simulink model "MPCfastmpc"  (R2023a)
settings: Solver=ode4  StartTime=0.0  StopTime=tsim  FixedStep=baseRate  RelTol=1e-6  AbsTol=1e-6
values from neighbouring files (symbols this model uses):
  Ad = -C(7:12,4:9)    [theFastMPCSolver3.m]
  ALGORITHM = 7    [Run_Initializer.m]
  con0 = [n*N, 2*N, N, N, N]    [Run_Initializer.m]
  Gamma1_el = 0.12    [Run_Initializer.m]
  Gamma1_sh = 0.005    [Run_Initializer.m]
  Gamma1_wr = 0.025    [Run_Initializer.m]
  Gamma2_el = 5    [Run_Initializer.m]
  Gamma2_sh = 5    [Run_Initializer.m]
  Gamma2_wr = 5    [Run_Initializer.m]
  Gamma3_el = 10    [Run_Initializer.m]
  Gamma3_sh = 40    [Run_Initializer.m]
  Gamma3_wr = 40    [Run_Initializer.m]
  Gamma4_el = 0.039    [Run_Initializer.m]
  Gamma4_sh = 0.015    [Run_Initializer.m]
  Gamma4_wr = 0.029    [Run_Initializer.m]
  Gamma5_el = 800    [Run_Initializer.m]
  Gamma5_sh = 800    [Run_Initializer.m]
  Gamma5_wr = 800    [Run_Initializer.m]
  Gamma6_el = 0.000001    (= 1e-06)    [Run_Initializer.m]
  Gamma6_sh = 0.005    [Run_Initializer.m]
  Gamma6_wr = 0.02    [Run_Initializer.m]
  init_states_BLACK = [ct;thetat0].'    [Run_Initializer.m]
  init_states_BLUE = [pobj1;0].'    [Run_Initializer.m]
  init_states_RED = xi(1:3).'    [Run_Initializer.m]
  Kd_elarm = 0.8    [Run_Initializer.m]
  Kd_sharm = 1.0    (= 1)    [Run_Initializer.m]
  Kd_wrarm = 0.6    [Run_Initializer.m]
  Kp_elarm = 1.2    [Run_Initializer.m]
  Kp_sharm = 1.5    [Run_Initializer.m]
  Kp_wrarm = 2    [Run_Initializer.m]
  maxiterations = 10    [Run_Initializer.m]
  N = 15    [Run_Initializer.m]    (also in theFastMPCSolver3.m = length(z)/9)
  n = size(b,1)    [theFastMPCSolver3.m]
  Phi = 2*H + kappa*P.'*d2*P    [theFastMPCSolver3.m]
  Td = 2    [Run_Initializer.m]
  thetat_dot = 2.5 * d2r    (= 0.0436332312999)    [Run_Initializer.m]
  tol = 0.00015    [Run_Initializer.m]
  Tz_lim_elarm = .1    (= 0.1)    [Run_Initializer.m]
  Tz_lim_sharm = .1    (= 0.1)    [Run_Initializer.m]
  Tz_lim_wrarm = .1    (= 0.1)    [Run_Initializer.m]
  vobj1 = [0.00;0.00]    [Run_Initializer.m]
  vtar = [-0.005;0.005]    [Run_Initializer.m]
undefined symbols (not defined in the file or in its folder): a1, a2, a3, b0, b1, b2, b3, baseRate, cdockdeltax, cdockoa, Cmat, DiscIntNeverNeededParam, drop_states_ARM, drop_states_BLACK, drop_states_BLUE, drop_states_RED, ecoa, F_Black_X_nominal, F_Black_Y_nominal, F_Blue_X_nominal, F_Blue_Y_nominal, F_red_X_nominal, F_red_Y_nominal, F_thrusters_BLACK, F_thrusters_BLUE, F_thrusters_RED, Fmat, gamma, H, IBLACK, IBLUE, IDIST, IEE, IPROX, IRED, Kd_tb, Kd_tblue, Kd_tr, Kd_xb, Kd_xblue, Kd_xr, Kd_yb, Kd_yblue, Kd_yr, KOZ_actual, Kp_tb, Kp_tblue, Kp_tr, Kp_xb, Kp_xblue, Kp_xr, Kp_yb, Kp_yblue, Kp_yr, mBLACK, mBLUE, mDIST, mEE, mPROX, mRED ... (+29)
libraries: nvidiaSharedBlocks x8, simulink x8, dspsigops x6, dspstat3 x5, MainLibrary x4
(part 6 of 10)

== system MPCfastmpc/Phase #3: Experiment/Change BLUE Behavior/Sub-Phase #1/Custom Discrete PD (Attitude) ==
  ez : Inport
  Sum3 : Sum
  kd_tb : Gain  Gain=Kd_tblue
  kp_tb : Gain  Gain=Kp_tblue
  "x_dot -> x1" : Subsystem
  Tz : Outport  VectorParamsAs1DForOutWhenUnconnected=off
  wires:
  kd_tb/1 -> Sum3/1
  Sum3/1 -> Tz/1
  kp_tb/1 -> Sum3/2
  "x_dot -> x1"/1(dy(t)/dt) -> kd_tb/1
  ez/1 -> "x_dot -> x1"/1(y(t)), kp_tb/1

== system MPCfastmpc/Phase #3: Experiment/Change BLUE Behavior/Sub-Phase #1/Custom Discrete PD (X-Position) ==
  ex : Inport
  Sum3 : Sum
  kd_xb : Gain  Gain=Kd_xblue
  kp_xb : Gain  Gain=Kp_xblue
  "x_dot -> x1" : Subsystem
  Fx : Outport  VectorParamsAs1DForOutWhenUnconnected=off
  wires:
  kd_xb/1 -> Sum3/1
  ex/1 -> "x_dot -> x1"/1(y(t)), kp_xb/1
  kp_xb/1 -> Sum3/2
  "x_dot -> x1"/1(dy(t)/dt) -> kd_xb/1
  Sum3/1 -> Fx/1

== system MPCfastmpc/Phase #3: Experiment/Change BLUE Behavior/Sub-Phase #1/Custom Discrete PD (Y-Position) ==
  ey : Inport
  Sum3 : Sum
  kd_yb : Gain  Gain=Kd_yblue
  kp_yb : Gain  Gain=Kp_yblue
  "x_dot -> x1" : Subsystem
  Fy : Outport  VectorParamsAs1DForOutWhenUnconnected=off
  wires:
  kd_yb/1 -> Sum3/1
  Sum3/1 -> Fy/1
  kp_yb/1 -> Sum3/2
  "x_dot -> x1"/1(dy(t)/dt) -> kd_yb/1
  ey/1 -> "x_dot -> x1"/1(y(t)), kp_yb/1

== system MPCfastmpc/Phase #3: Experiment/Change BLUE Behavior/Sub-Phase #1/Hough Control ==
  Ref : Inport
  Act : Inport  Port=2
  MATLAB Function2 : MATLAB Function  TreatAsAtomicUnit=on
  MATLAB Function3 : MATLAB Function  TreatAsAtomicUnit=on
  MATLAB Function4 : MATLAB Function  TreatAsAtomicUnit=on
  Subtract2 : Sum  Inputs=+-
  Err : Outport  VectorParamsAs1DForOutWhenUnconnected=off
  wires:
  MATLAB Function4/1(e_out) -> Err/1
  MATLAB Function2/1(Oy) -> MATLAB Function4/1(Oy)
  Subtract2/1 -> MATLAB Function4/2(e_in)
  MATLAB Function2/2(Ox) -> Subtract2/1
  Act/1 -> MATLAB Function3/1(z)
  Ref/1 -> MATLAB Function2/1(z)
  MATLAB Function3/1(Ox) -> Subtract2/2

== system MPCfastmpc/Phase #3: Experiment/Change BLUE Behavior/Sub-Phase #2 /Custom Discrete PD (Attitude) ==
  ez : Inport
  Sum3 : Sum
  kd_tb : Gain  Gain=Kd_tblue
  kp_tb : Gain  Gain=Kp_tblue
  "x_dot -> x1" : Subsystem
  Tz : Outport  VectorParamsAs1DForOutWhenUnconnected=off
  wires:
  kd_tb/1 -> Sum3/1
  Sum3/1 -> Tz/1
  kp_tb/1 -> Sum3/2
  "x_dot -> x1"/1(dy(t)/dt) -> kd_tb/1
  ez/1 -> "x_dot -> x1"/1(y(t)), kp_tb/1

== system MPCfastmpc/Phase #3: Experiment/Change BLUE Behavior/Sub-Phase #2 /Custom Discrete PD (X-Position) ==
  ex : Inport
  Sum3 : Sum
  kd_xb : Gain  Gain=Kd_xblue
  kp_xb : Gain  Gain=Kp_xblue
  "x_dot -> x1" : Subsystem
  Fx : Outport  VectorParamsAs1DForOutWhenUnconnected=off
  wires:
  kd_xb/1 -> Sum3/1
  ex/1 -> "x_dot -> x1"/1(y(t)), kp_xb/1
  kp_xb/1 -> Sum3/2
  "x_dot -> x1"/1(dy(t)/dt) -> kd_xb/1
  Sum3/1 -> Fx/1

== system MPCfastmpc/Phase #3: Experiment/Change BLUE Behavior/Sub-Phase #2 /Custom Discrete PD (Y-Position) ==
  ey : Inport
  Sum3 : Sum
  kd_yb : Gain  Gain=Kd_yblue
  kp_yb : Gain  Gain=Kp_yblue
  "x_dot -> x1" : Subsystem
  Fy : Outport  VectorParamsAs1DForOutWhenUnconnected=off
  wires:
  kd_yb/1 -> Sum3/1
  Sum3/1 -> Fy/1
  kp_yb/1 -> Sum3/2
  "x_dot -> x1"/1(dy(t)/dt) -> kd_yb/1
  ey/1 -> "x_dot -> x1"/1(y(t)), kp_yb/1

== system MPCfastmpc/Phase #3: Experiment/Change BLUE Behavior/Sub-Phase #2 /Hough Control ==
  Ref : Inport
  Act : Inport  Port=2
  MATLAB Function2 : MATLAB Function  TreatAsAtomicUnit=on
  MATLAB Function3 : MATLAB Function  TreatAsAtomicUnit=on
  MATLAB Function4 : MATLAB Function  TreatAsAtomicUnit=on
  Subtract2 : Sum  Inputs=+-
  Err : Outport  VectorParamsAs1DForOutWhenUnconnected=off
  wires:
  MATLAB Function4/1(e_out) -> Err/1
  MATLAB Function2/1(Oy) -> MATLAB Function4/1(Oy)
  Subtract2/1 -> MATLAB Function4/2(e_in)
  MATLAB Function2/2(Ox) -> Subtract2/1
  Act/1 -> MATLAB Function3/1(z)
  Ref/1 -> MATLAB Function2/1(z)
  MATLAB Function3/1(Ox) -> Subtract2/2

== system MPCfastmpc/Phase #3: Experiment/Change BLUE Behavior/Sub-Phase #3 /Custom Discrete PD (Attitude) ==
  ez : Inport
  Sum3 : Sum
  kd_tb : Gain  Gain=Kd_tblue
  kp_tb : Gain  Gain=Kp_tblue
  "x_dot -> x1" : Subsystem
  Tz : Outport  VectorParamsAs1DForOutWhenUnconnected=off
  wires:
  kd_tb/1 -> Sum3/1
  Sum3/1 -> Tz/1
  kp_tb/1 -> Sum3/2
  "x_dot -> x1"/1(dy(t)/dt) -> kd_tb/1
  ez/1 -> "x_dot -> x1"/1(y(t)), kp_tb/1

== system MPCfastmpc/Phase #3: Experiment/Change BLUE Behavior/Sub-Phase #3 /Custom Discrete PD (X-Position) ==
  ex : Inport
  Sum3 : Sum
  kd_xb : Gain  Gain=Kd_xblue
  kp_xb : Gain  Gain=Kp_xblue
  "x_dot -> x1" : Subsystem
  Fx : Outport  VectorParamsAs1DForOutWhenUnconnected=off
  wires:
  kd_xb/1 -> Sum3/1
  ex/1 -> "x_dot -> x1"/1(y(t)), kp_xb/1
  kp_xb/1 -> Sum3/2
  "x_dot -> x1"/1(dy(t)/dt) -> kd_xb/1
  Sum3/1 -> Fx/1

== system MPCfastmpc/Phase #3: Experiment/Change BLUE Behavior/Sub-Phase #3 /Custom Discrete PD (Y-Position) ==
  ey : Inport
  Sum3 : Sum
  kd_yb : Gain  Gain=Kd_yblue
  kp_yb : Gain  Gain=Kp_yblue
  "x_dot -> x1" : Subsystem
  Fy : Outport  VectorParamsAs1DForOutWhenUnconnected=off
  wires:
  kd_yb/1 -> Sum3/1
  Sum3/1 -> Fy/1
  kp_yb/1 -> Sum3/2
  "x_dot -> x1"/1(dy(t)/dt) -> kd_yb/1
  ey/1 -> "x_dot -> x1"/1(y(t)), kp_yb/1

== system MPCfastmpc/Phase #3: Experiment/Change BLUE Behavior/Sub-Phase #3 /Hough Control ==
  Ref : Inport
  Act : Inport  Port=2
  MATLAB Function2 : MATLAB Function  TreatAsAtomicUnit=on
  MATLAB Function3 : MATLAB Function  TreatAsAtomicUnit=on
  MATLAB Function4 : MATLAB Function  TreatAsAtomicUnit=on
  Subtract2 : Sum  Inputs=+-
  Err : Outport  VectorParamsAs1DForOutWhenUnconnected=off
  wires:
  MATLAB Function4/1(e_out) -> Err/1
  MATLAB Function2/1(Oy) -> MATLAB Function4/1(Oy)
  Subtract2/1 -> MATLAB Function4/2(e_in)
  MATLAB Function2/2(Ox) -> Subtract2/1
  Act/1 -> MATLAB Function3/1(z)
  Ref/1 -> MATLAB Function2/1(z)
  MATLAB Function3/1(Ox) -> Subtract2/2

== system MPCfastmpc/Phase #3: Experiment/Change BLUE Behavior/Sub-Phase #3 /Subsystem ==
  Add : Sum
  Add1 : Sum  Inputs=+-
  Constant : Constant  Value=vobj1
  Constant1 : Constant  Value=init_states_BLUE(1)
  Constant2 : Constant  Value=Phase3_SubPhase2_End
  Data Store Read : DataStoreRead  DataStoreName=Univ_Time  IndexOptions=Index vector (dialog)  Indices=1  OutputSizes=1
  Demux : Demux  Outputs=2
  Product : Product
  Terminator : Terminator
  Out1 : Outport
  wires:
  Add/1 -> Out1/1
  Demux/2 -> Terminator/1
  Constant/1 -> Demux/1
  Constant1/1 -> Add/1
  Product/1 -> Add/2
  Demux/1 -> Product/1
  Constant2/1 -> Add1/2
  Data Store Read/1 -> Add1/1
  Add1/1 -> Product/2

== system MPCfastmpc/Phase #3: Experiment/Change BLUE Behavior/Sub-Phase #3 /Subsystem1 ==
  Add : Sum
  Add1 : Sum  Inputs=+-
  Constant : Constant  Value=vobj1
  Constant1 : Constant  Value=init_states_BLUE(2)
  Constant2 : Constant  Value=Phase3_SubPhase2_End
  Data Store Read : DataStoreRead  DataStoreName=Univ_Time  IndexOptions=Index vector (dialog)  Indices=1  OutputSizes=1
  Demux : Demux  Outputs=2
  Product : Product
  Terminator : Terminator
  Out1 : Outport
  wires:
  Add/1 -> Out1/1
  Constant/1 -> Demux/1
  Constant1/1 -> Add/1
  Product/1 -> Add/2
  Constant2/1 -> Add1/2
  Data Store Read/1 -> Add1/1
  Add1/1 -> Product/2
  Demux/1 -> Terminator/1
  Demux/2 -> Product/1

== system MPCfastmpc/Phase #3: Experiment/Change BLUE Behavior/Sub-Phase #4/Custom Discrete PD (Attitude) ==
  ez : Inport
  Sum3 : Sum
  kd_tb : Gain  Gain=Kd_tblue
  kp_tb : Gain  Gain=Kp_tblue
  "x_dot -> x1" : Subsystem
  Tz : Outport  VectorParamsAs1DForOutWhenUnconnected=off
  wires:
  kd_tb/1 -> Sum3/1
  Sum3/1 -> Tz/1
  kp_tb/1 -> Sum3/2
  "x_dot -> x1"/1(dy(t)/dt) -> kd_tb/1
  ez/1 -> "x_dot -> x1"/1(y(t)), kp_tb/1

== system MPCfastmpc/Phase #3: Experiment/Change BLUE Behavior/Sub-Phase #4/Custom Discrete PD (X-Position) ==
  ex : Inport
  Sum3 : Sum
  kd_xb : Gain  Gain=Kd_xblue
  kp_xb : Gain  Gain=Kp_xblue
  "x_dot -> x1" : Subsystem
  Fx : Outport  VectorParamsAs1DForOutWhenUnconnected=off
  wires:
  kd_xb/1 -> Sum3/1
  ex/1 -> "x_dot -> x1"/1(y(t)), kp_xb/1
  kp_xb/1 -> Sum3/2
  "x_dot -> x1"/1(dy(t)/dt) -> kd_xb/1
  Sum3/1 -> Fx/1

== system MPCfastmpc/Phase #3: Experiment/Change BLUE Behavior/Sub-Phase #4/Custom Discrete PD (Y-Position) ==
  ey : Inport
  Sum3 : Sum
  kd_yb : Gain  Gain=Kd_yblue
  kp_yb : Gain  Gain=Kp_yblue
  "x_dot -> x1" : Subsystem
  Fy : Outport  VectorParamsAs1DForOutWhenUnconnected=off
  wires:
  kd_yb/1 -> Sum3/1
  Sum3/1 -> Fy/1
  kp_yb/1 -> Sum3/2
  "x_dot -> x1"/1(dy(t)/dt) -> kd_yb/1
  ey/1 -> "x_dot -> x1"/1(y(t)), kp_yb/1

== system MPCfastmpc/Phase #3: Experiment/Change BLUE Behavior/Sub-Phase #4/Hough Control ==
  Ref : Inport
  Act : Inport  Port=2
  MATLAB Function2 : MATLAB Function  TreatAsAtomicUnit=on
  MATLAB Function3 : MATLAB Function  TreatAsAtomicUnit=on
  MATLAB Function4 : MATLAB Function  TreatAsAtomicUnit=on
  Subtract2 : Sum  Inputs=+-
  Err : Outport  VectorParamsAs1DForOutWhenUnconnected=off
  wires:
  MATLAB Function4/1(e_out) -> Err/1
  MATLAB Function2/1(Oy) -> MATLAB Function4/1(Oy)
  Subtract2/1 -> MATLAB Function4/2(e_in)
  MATLAB Function2/2(Ox) -> Subtract2/1
  Act/1 -> MATLAB Function3/1(z)
  Ref/1 -> MATLAB Function2/1(z)
  MATLAB Function3/1(Ox) -> Subtract2/2

== system MPCfastmpc/Phase #3: Experiment/Change BLUE Behavior/Sub-Phase #4/Subsystem ==
  Add : Sum
  Add1 : Sum  Inputs=+-
  Constant : Constant  Value=vobj1
  Constant1 : Constant  Value=init_states_BLUE(1)
  Constant2 : Constant  Value=Phase3_SubPhase2_End
  Data Store Read : DataStoreRead  DataStoreName=Univ_Time  IndexOptions=Index vector (dialog)  Indices=1  OutputSizes=1
  Demux : Demux  Outputs=2
  Product : Product
  Terminator : Terminator
  Out1 : Outport
  wires:
  Add/1 -> Out1/1
  Demux/2 -> Terminator/1
  Constant/1 -> Demux/1
  Constant1/1 -> Add/1
  Product/1 -> Add/2
  Demux/1 -> Product/1
  Constant2/1 -> Add1/2
  Data Store Read/1 -> Add1/1
  Add1/1 -> Product/2

== system MPCfastmpc/Phase #3: Experiment/Change BLUE Behavior/Sub-Phase #4/Subsystem1 ==
  Add : Sum
  Add1 : Sum  Inputs=+-
  Constant : Constant  Value=vobj1
  Constant1 : Constant  Value=init_states_BLUE(2)
  Constant2 : Constant  Value=Phase3_SubPhase2_End
  Data Store Read : DataStoreRead  DataStoreName=Univ_Time  IndexOptions=Index vector (dialog)  Indices=1  OutputSizes=1
  Demux : Demux  Outputs=2
  Product : Product
  Terminator : Terminator
  Out1 : Outport
  wires:
  Add/1 -> Out1/1
  Constant/1 -> Demux/1
  Constant1/1 -> Add/1
  Product/1 -> Add/2
  Constant2/1 -> Add1/2
  Data Store Read/1 -> Add1/1
  Add1/1 -> Product/2
  Demux/1 -> Terminator/1
  Demux/2 -> Product/1

== system MPCfastmpc/Phase #3: Experiment/Change RED Behavior/Sub-Phase #1/Custom Discrete PD (Attitude) ==
  ez : Inport
  Sum3 : Sum
  kd_tr : Gain  Gain=Kd_tr
  kp_tr : Gain  Gain=Kp_tr
  "x_dot -> x2" : Subsystem
  Tz : Outport  VectorParamsAs1DForOutWhenUnconnected=off
  wires:
  kd_tr/1 -> Sum3/1
  Sum3/1 -> Tz/1
  kp_tr/1 -> Sum3/2
  "x_dot -> x2"/1(dy(t)/dt) -> kd_tr/1
  ez/1 -> "x_dot -> x2"/1(y(t)), kp_tr/1

== system MPCfastmpc/Phase #3: Experiment/Change RED Behavior/Sub-Phase #1/Custom Discrete PD (X-Position) ==
  ex : Inport
  Sum3 : Sum
  kd_xr : Gain  Gain=Kd_xr
  kp_xr : Gain  Gain=Kp_xr
  "x_dot -> x2" : Subsystem
  Fx : Outport  VectorParamsAs1DForOutWhenUnconnected=off
  wires:
  kd_xr/1 -> Sum3/1
  ex/1 -> "x_dot -> x2"/1(y(t)), kp_xr/1
  kp_xr/1 -> Sum3/2
  "x_dot -> x2"/1(dy(t)/dt) -> kd_xr/1
  Sum3/1 -> Fx/1

== system MPCfastmpc/Phase #3: Experiment/Change RED Behavior/Sub-Phase #1/Custom Discrete PD (Y-Position) ==
  ey : Inport
  Sum3 : Sum
  kd_yr : Gain  Gain=Kd_yr
  kp_yr : Gain  Gain=Kp_yr
  "x_dot -> x2" : Subsystem
  Fy : Outport  VectorParamsAs1DForOutWhenUnconnected=off
  wires:
  kd_yr/1 -> Sum3/1
  Sum3/1 -> Fy/1
  kp_yr/1 -> Sum3/2
  "x_dot -> x2"/1(dy(t)/dt) -> kd_yr/1
  ey/1 -> "x_dot -> x2"/1(y(t)), kp_yr/1

== system MPCfastmpc/Phase #3: Experiment/Change RED Behavior/Sub-Phase #1/Hough Control ==
  Ref : Inport
  Act : Inport  Port=2
  MATLAB Function2 : MATLAB Function  TreatAsAtomicUnit=on
  MATLAB Function3 : MATLAB Function  TreatAsAtomicUnit=on
  MATLAB Function4 : MATLAB Function  TreatAsAtomicUnit=on
  Subtract2 : Sum  Inputs=+-
  Err : Outport  VectorParamsAs1DForOutWhenUnconnected=off
  wires:
  MATLAB Function4/1(e_out) -> Err/1
  MATLAB Function2/1(Oy) -> MATLAB Function4/1(Oy)
  Subtract2/1 -> MATLAB Function4/2(e_in)
  MATLAB Function2/2(Ox) -> Subtract2/1
  Act/1 -> MATLAB Function3/1(z)
  Ref/1 -> MATLAB Function2/1(z)
  MATLAB Function3/1(Ox) -> Subtract2/2

== system MPCfastmpc/Phase #3: Experiment/Change RED Behavior/Sub-Phase #1/RED+ARM ==
  note: ARM Control Law - RED
  note: This section is reserved for any control law for the robotic manipulator.
  Action Port : ActionPort
  Constant4 : Constant  Value=pi/2
  Constant5 : Constant  Value=pi/2
  Constant6 : Constant  Value=0
  Constant7 : Constant
  Data Store Read1 : DataStoreRead  DataStoreName=isSim  IndexOptions=Index vector (dialog)  Indices=1  OutputSizes=1
  Data Store Write : DataStoreWrite  DataStoreName=RED_Shoulder_Command  IndexOptions=Index vector (dialog)  Indices=1  OutputSizes=1
  Data Store Write1 : DataStoreWrite  DataStoreName=RED_Elbow_Command  IndexOptions=Index vector (dialog)  Indices=1  OutputSizes=1
  Data Store Write2 : DataStoreWrite  DataStoreName=RED_Wrist_Command  IndexOptions=Index vector (dialog)  Indices=1  OutputSizes=1
  Data Store Write3 : DataStoreWrite  DataStoreName=RED_ARM_Control_Mode  IndexOptions=Index vector (dialog)  Indices=1  OutputSizes=1
  "If 'simMode' set to '1', then this is a simulation and the dynamics will be simulated. Otherwise, this is an experiment, and the simulation will not be run." : If  IfExpression=u1 == 1
  Merge : Merge
  Merge1 : Merge
  Merge2 : Merge
  Passthrough for Experiment : Subsystem  TreatAsAtomicUnit=on
  Simulated Position Controller : Subsystem  TreatAsAtomicUnit=on
  wires:
  Constant7/1 -> Data Store Write3/1
  Constant6/1 -> Passthrough for Experiment/3(q3_desired), Simulated Position Controller/3(q3_desired)
  Constant4/1 -> Passthrough for Experiment/1(q1_desired), Simulated Position Controller/1(q1_desired)
  Constant5/1 -> Passthrough for Experiment/2(q2_desired), Simulated Position Controller/2(q2_desired)
  Data Store Read1/1 -> "If 'simMode' set to '1', then this is a simulation and the dynamics will be simulated. Otherwise, this is an experiment, and the simulation will not be run."/1
  "If 'simMode' set to '1', then this is a simulation and the dynamics will be simulated. Otherwise, this is an experiment, and the simulation will not be run."/1 -> Simulated Position Controller/Action
  "If 'simMode' set to '1', then this is a simulation and the dynamics will be simulated. Otherwise, this is an experiment, and the simulation will not be run."/2 -> Passthrough for Experiment/Action
  Simulated Position Controller/1(q1_command) -> Merge/1
  Passthrough for Experiment/1(q1_command) -> Merge/2
  Merge/1 -> Data Store Write/1
  Simulated Position Controller/2(q2_command) -> Merge1/1
  Merge1/1 -> Data Store Write1/1
  Passthrough for Experiment/2(q2_command) -> Merge1/2
  Simulated Position Controller/3(q3_command) -> Merge2/1
  Passthrough for Experiment/3(q3_command) -> Merge2/2
  Merge2/1 -> Data Store Write2/1

== system MPCfastmpc/Phase #3: Experiment/Change RED Behavior/Sub-Phase #2 /RED+ARM ==
  note: ARM Control Law - RED
  note: This section is reserved for any control law for the robotic manipulator.
  Action Port : ActionPort
  Constant4 : Constant  Value=pi/2
  Constant5 : Constant  Value=pi/2
  Constant6 : Constant  Value=0
  Constant7 : Constant
  Data Store Read1 : DataStoreRead  DataStoreName=isSim  IndexOptions=Index vector (dialog)  Indices=1  OutputSizes=1
  Data Store Write : DataStoreWrite  DataStoreName=RED_Shoulder_Command  IndexOptions=Index vector (dialog)  Indices=1  OutputSizes=1
  Data Store Write1 : DataStoreWrite  DataStoreName=RED_Elbow_Command  IndexOptions=Index vector (dialog)  Indices=1  OutputSizes=1
  Data Store Write2 : DataStoreWrite  DataStoreName=RED_Wrist_Command  IndexOptions=Index vector (dialog)  Indices=1  OutputSizes=1
  Data Store Write3 : DataStoreWrite  DataStoreName=RED_ARM_Control_Mode  IndexOptions=Index vector (dialog)  Indices=1  OutputSizes=1
  "If 'simMode' set to '1', then this is a simulation and the dynamics will be simulated. Otherwise, this is an experiment, and the simulation will not be run." : If  IfExpression=u1 == 1
  Merge : Merge
  Merge1 : Merge
  Merge2 : Merge
  Passthrough for Experiment : Subsystem  TreatAsAtomicUnit=on
  Simulated Position Controller : Subsystem  TreatAsAtomicUnit=on
  wires:
  Constant7/1 -> Data Store Write3/1
  Constant6/1 -> Passthrough for Experiment/3(q3_desired), Simulated Position Controller/3(q3_desired)
  Constant4/1 -> Passthrough for Experiment/1(q1_desired), Simulated Position Controller/1(q1_desired)
  Constant5/1 -> Passthrough for Experiment/2(q2_desired), Simulated Position Controller/2(q2_desired)
  Data Store Read1/1 -> "If 'simMode' set to '1', then this is a simulation and the dynamics will be simulated. Otherwise, this is an experiment, and the simulation will not be run."/1
  "If 'simMode' set to '1', then this is a simulation and the dynamics will be simulated. Otherwise, this is an experiment, and the simulation will not be run."/1 -> Simulated Position Controller/Action
  "If 'simMode' set to '1', then this is a simulation and the dynamics will be simulated. Otherwise, this is an experiment, and the simulation will not be run."/2 -> Passthrough for Experiment/Action
  Simulated Position Controller/1(q1_command) -> Merge/1
  Passthrough for Experiment/1(q1_command) -> Merge/2
  Merge/1 -> Data Store Write/1
  Simulated Position Controller/2(q2_command) -> Merge1/1
  Merge1/1 -> Data Store Write1/1
  Passthrough for Experiment/2(q2_command) -> Merge1/2
  Simulated Position Controller/3(q3_command) -> Merge2/1
  Passthrough for Experiment/3(q3_command) -> Merge2/2
  Merge2/1 -> Data Store Write2/1

== system MPCfastmpc/Phase #3: Experiment/Change RED Behavior/Sub-Phase #3 /RED+ARM ==
  note: ARM Control Law - RED
  note: This section is reserved for any control law for the robotic manipulator.
  Action Port : ActionPort
  Constant4 : Constant  Value=pi/2
  Constant5 : Constant  Value=pi/2
  Constant6 : Constant  Value=0
  Constant7 : Constant
  Data Store Read1 : DataStoreRead  DataStoreName=isSim  IndexOptions=Index vector (dialog)  Indices=1  OutputSizes=1
  Data Store Write : DataStoreWrite  DataStoreName=RED_Shoulder_Command  IndexOptions=Index vector (dialog)  Indices=1  OutputSizes=1
  Data Store Write1 : DataStoreWrite  DataStoreName=RED_Elbow_Command  IndexOptions=Index vector (dialog)  Indices=1  OutputSizes=1
  Data Store Write2 : DataStoreWrite  DataStoreName=RED_Wrist_Command  IndexOptions=Index vector (dialog)  Indices=1  OutputSizes=1
  Data Store Write3 : DataStoreWrite  DataStoreName=RED_ARM_Control_Mode  IndexOptions=Index vector (dialog)  Indices=1  OutputSizes=1
  "If 'simMode' set to '1', then this is a simulation and the dynamics will be simulated. Otherwise, this is an experiment, and the simulation will not be run." : If  IfExpression=u1 == 1
  Merge : Merge
  Merge1 : Merge
  Merge2 : Merge
  Passthrough for Experiment : Subsystem  TreatAsAtomicUnit=on
  Simulated Position Controller : Subsystem  TreatAsAtomicUnit=on
  wires:
  Constant7/1 -> Data Store Write3/1
  Constant6/1 -> Passthrough for Experiment/3(q3_desired), Simulated Position Controller/3(q3_desired)
  Constant4/1 -> Passthrough for Experiment/1(q1_desired), Simulated Position Controller/1(q1_desired)
  Constant5/1 -> Passthrough for Experiment/2(q2_desired), Simulated Position Controller/2(q2_desired)
  Data Store Read1/1 -> "If 'simMode' set to '1', then this is a simulation and the dynamics will be simulated. Otherwise, this is an experiment, and the simulation will not be run."/1
  "If 'simMode' set to '1', then this is a simulation and the dynamics will be simulated. Otherwise, this is an experiment, and the simulation will not be run."/1 -> Simulated Position Controller/Action
  "If 'simMode' set to '1', then this is a simulation and the dynamics will be simulated. Otherwise, this is an experiment, and the simulation will not be run."/2 -> Passthrough for Experiment/Action
  Simulated Position Controller/1(q1_command) -> Merge/1
  Passthrough for Experiment/1(q1_command) -> Merge/2
  Merge/1 -> Data Store Write/1
  Simulated Position Controller/2(q2_command) -> Merge1/1
  Merge1/1 -> Data Store Write1/1
  Passthrough for Experiment/2(q2_command) -> Merge1/2
  Simulated Position Controller/3(q3_command) -> Merge2/1
  Passthrough for Experiment/3(q3_command) -> Merge2/2
  Merge2/1 -> Data Store Write2/1

== system MPCfastmpc/Phase #3: Experiment/Change RED Behavior/Sub-Phase #4/RED+ARM ==
  note: ARM Control Law - RED
  note: This section is reserved for any control law for the robotic manipulator.
  Action Port : ActionPort
  1-D Lookup Table : Lookup_n-D  NumberOfTableDimensions=1  BreakpointsForDimension1=[0 Phase3_SubPhase4_Duration]  Table=[pi/2 pi/3]  InternalRulePriority=Speed  RndMeth=Simplest
  Constant1 : Constant  Value=Phase3_SubPhase3_End
  Constant6 : Constant  Value=0
  Constant7 : Constant
  Data Store Read : DataStoreRead  DataStoreName=Univ_Time  IndexOptions=Index vector (dialog)  Indices=1  OutputSizes=1
  Data Store Read1 : DataStoreRead  DataStoreName=isSim  IndexOptions=Index vector (dialog)  Indices=1  OutputSizes=1
  Data Store Write : DataStoreWrite  DataStoreName=RED_Shoulder_Command  IndexOptions=Index vector (dialog)  Indices=1  OutputSizes=1
  Data Store Write1 : DataStoreWrite  DataStoreName=RED_Elbow_Command  IndexOptions=Index vector (dialog)  Indices=1  OutputSizes=1
  Data Store Write2 : DataStoreWrite  DataStoreName=RED_Wrist_Command  IndexOptions=Index vector (dialog)  Indices=1  OutputSizes=1
  Data Store Write3 : DataStoreWrite  DataStoreName=RED_ARM_Control_Mode  IndexOptions=Index vector (dialog)  Indices=1  OutputSizes=1
  "If 'simMode' set to '1', then this is a simulation and the dynamics will be simulated. Otherwise, this is an experiment, and the simulation will not be run." : If  IfExpression=u1 == 1
  Merge : Merge
  Merge1 : Merge
  Merge2 : Merge
  Passthrough for Experiment : Subsystem  TreatAsAtomicUnit=on
  Simulated Position Controller : Subsystem  TreatAsAtomicUnit=on
  Subtract : Sum  Inputs=+-
  wires:
  Constant7/1 -> Data Store Write3/1
  Constant6/1 -> Passthrough for Experiment/3(q3_desired), Simulated Position Controller/3(q3_desired)
  1-D Lookup Table/1 -> Passthrough for Experiment/2(q2_desired), Simulated Position Controller/2(q2_desired), Passthrough for Experiment/1(q1_desired), Simulated Position Controller/1(q1_desired)
  Data Store Read1/1 -> "If 'simMode' set to '1', then this is a simulation and the dynamics will be simulated. Otherwise, this is an experiment, and the simulation will not be run."/1
  "If 'simMode' set to '1', then this is a simulation and the dynamics will be simulated. Otherwise, this is an experiment, and the simulation will not be run."/1 -> Simulated Position Controller/Action
  "If 'simMode' set to '1', then this is a simulation and the dynamics will be simulated. Otherwise, this is an experiment, and the simulation will not be run."/2 -> Passthrough for Experiment/Action
  Simulated Position Controller/1(q1_command) -> Merge/1
  Passthrough for Experiment/1(q1_command) -> Merge/2
  Merge/1 -> Data Store Write/1
  Simulated Position Controller/2(q2_command) -> Merge1/1
  Merge1/1 -> Data Store Write1/1
  Passthrough for Experiment/2(q2_command) -> Merge1/2
  Simulated Position Controller/3(q3_command) -> Merge2/1
  Passthrough for Experiment/3(q3_command) -> Merge2/2
  Merge2/1 -> Data Store Write2/1
  Subtract/1 -> 1-D Lookup Table/1
  Constant1/1 -> Subtract/2
  Data Store Read/1 -> Subtract/1

== system MPCfastmpc/Phase #3: Experiment/Change RED Behavior/Sub-Phase #4/Subsystem ==
  Data Store Read : DataStoreRead  DataStoreName=RED_Rz  IndexOptions=Index vector (dialog)  Indices=1  OutputSizes=1
  Data Store Read1 : DataStoreRead  DataStoreName=RED_Rev_Counter  IndexOptions=Index vector (dialog)  Indices=1  OutputSizes=1
  Data Store Read2 : DataStoreRead  DataStoreName=BLACK_Rz  IndexOptions=Index vector (dialog)  Indices=1  OutputSizes=1
  Data Store Read3 : DataStoreRead  DataStoreName=BLACK_Rev_Counter  IndexOptions=Index vector (dialog)  Indices=1  OutputSizes=1
  Data Store Write : DataStoreWrite  DataStoreName=RED_Rev_Counter  IndexOptions=Index vector (dialog)  Indices=1  OutputSizes=1
  Data Store Write1 : DataStoreWrite  DataStoreName=RED_Rz_Cont  IndexOptions=Index vector (dialog)  Indices=1  OutputSizes=1
  Data Store Write2 : DataStoreWrite  DataStoreName=BLACK_Rev_Counter  IndexOptions=Index vector (dialog)  Indices=1  OutputSizes=1
  Data Store Write3 : DataStoreWrite  DataStoreName=BLACK_Rz_Cont  IndexOptions=Index vector (dialog)  Indices=1  OutputSizes=1
  Delay : Delay  DelayLength=1
  Delay1 : Delay  DelayLength=1
  MATLAB Function : MATLAB Function  TreatAsAtomicUnit=on
  MATLAB Function1 : MATLAB Function  TreatAsAtomicUnit=on
  MATLAB Function2 : MATLAB Function  TreatAsAtomicUnit=on
  MATLAB Function3 : MATLAB Function  TreatAsAtomicUnit=on
  wires:
  Delay/1 -> MATLAB Function1/2(theta_psm1)
  MATLAB Function/1(x) -> Delay/1, MATLAB Function1/1(theta_ps)
  Data Store Read/1 -> MATLAB Function/1("x ")
  Data Store Read1/1 -> MATLAB Function1/3("revcounter ")
  MATLAB Function1/2(revcounter) -> Data Store Write/1
  MATLAB Function1/1(theta_cont) -> Data Store Write1/1
  Data Store Read3/1 -> MATLAB Function3/3("revcounter ")
  MATLAB Function3/2(revcounter) -> Data Store Write2/1
  Data Store Read2/1 -> MATLAB Function2/1("x ")
  Delay1/1 -> MATLAB Function3/2(theta_psm1)
  MATLAB Function3/1(theta_cont) -> Data Store Write3/1
  MATLAB Function2/1(x) -> Delay1/1, MATLAB Function3/1(theta_ps)

== system MPCfastmpc/Phase #4: Return Home/Change RED Behavior/RED+ARM/Passthrough for Experiment ==
  q1_desired : Inport
  q2_desired : Inport  Port=2
  q3_desired : Inport  Port=3
  Action Port : ActionPort
  q1_command : Outport
  q2_command : Outport  Port=2
  q3_command : Outport  Port=3
  wires:
  q3_desired/1 -> q3_command/1
  q1_desired/1 -> q1_command/1
  q2_desired/1 -> q2_command/1

== system MPCfastmpc/Phase #4: Return Home/Change RED Behavior/RED+ARM/Simulated Position Controller ==
  q1_desired : Inport
  q2_desired : Inport  Port=2
  q3_desired : Inport  Port=3
  Action Port : ActionPort
  Custom Discrete PD (Elbow) : Subsystem
  Custom Discrete PD (Shoulder) : Subsystem
  Custom Discrete PD (Wrist) : Subsystem
  Data Store Read : DataStoreRead  DataStoreName=RED_Rz_Shoulder  IndexOptions=Index vector (dialog)  Indices=1  OutputSizes=1
  Data Store Read5 : DataStoreRead  DataStoreName=RED_Rz_Elbow  IndexOptions=Index vector (dialog)  Indices=1  OutputSizes=1
  Data Store Read6 : DataStoreRead  DataStoreName=RED_Rz_Wrist  IndexOptions=Index vector (dialog)  Indices=1  OutputSizes=1
  Saturation : Saturate  UpperLimit=Tz_lim_sharm  LowerLimit=-Tz_lim_sharm
  Saturation1 : Saturate  UpperLimit=Tz_lim_elarm  LowerLimit=-Tz_lim_elarm
  Saturation3 : Saturate  UpperLimit=Tz_lim_wrarm  LowerLimit=-Tz_lim_wrarm
  Subtract2 : Sum  Inputs=+-
  Subtract3 : Sum  Inputs=+-
  Subtract4 : Sum  Inputs=+-
  q1_command : Outport
  q2_command : Outport  Port=2
  q3_command : Outport  Port=3
  wires:
  Saturation3/1 -> q3_command/1
  Subtract4/1 -> Custom Discrete PD (Wrist)/1(ey)
  Custom Discrete PD (Shoulder)/1(Fx) -> Saturation/1
  Custom Discrete PD (Elbow)/1(Fy) -> Saturation1/1
  Saturation/1 -> q1_command/1
  Subtract2/1 -> Custom Discrete PD (Shoulder)/1(ex)
  Saturation1/1 -> q2_command/1
  Custom Discrete PD (Wrist)/1(Fy) -> Saturation3/1
  Subtract3/1 -> Custom Discrete PD (Elbow)/1(ey)
  Data Store Read/1 -> Subtract2/2
  Data Store Read5/1 -> Subtract3/2
  Data Store Read6/1 -> Subtract4/2
  q1_desired/1 -> Subtract2/1
  q2_desired/1 -> Subtract3/1
  q3_desired/1 -> Subtract4/1

== system MPCfastmpc/Phase #5: Hold Home/Change RED Behavior/RED+ARM/Passthrough for Experiment ==
  q1_desired : Inport
  q2_desired : Inport  Port=2
  q3_desired : Inport  Port=3
  Action Port : ActionPort
  q1_command : Outport
  q2_command : Outport  Port=2
  q3_command : Outport  Port=3
  wires:
  q3_desired/1 -> q3_command/1
  q1_desired/1 -> q1_command/1
  q2_desired/1 -> q2_command/1

== system MPCfastmpc/Phase #5: Hold Home/Change RED Behavior/RED+ARM/Simulated Position Controller ==
  q1_desired : Inport
  q2_desired : Inport  Port=2
  q3_desired : Inport  Port=3
  Action Port : ActionPort
  Custom Discrete PD (Elbow) : Subsystem
  Custom Discrete PD (Shoulder) : Subsystem
  Custom Discrete PD (Wrist) : Subsystem
  Data Store Read : DataStoreRead  DataStoreName=RED_Rz_Shoulder  IndexOptions=Index vector (dialog)  Indices=1  OutputSizes=1
  Data Store Read5 : DataStoreRead  DataStoreName=RED_Rz_Elbow  IndexOptions=Index vector (dialog)  Indices=1  OutputSizes=1
  Data Store Read6 : DataStoreRead  DataStoreName=RED_Rz_Wrist  IndexOptions=Index vector (dialog)  Indices=1  OutputSizes=1
  Saturation : Saturate  UpperLimit=Tz_lim_sharm  LowerLimit=-Tz_lim_sharm
  Saturation1 : Saturate  UpperLimit=Tz_lim_elarm  LowerLimit=-Tz_lim_elarm
  Saturation3 : Saturate  UpperLimit=Tz_lim_wrarm  LowerLimit=-Tz_lim_wrarm
  Subtract2 : Sum  Inputs=+-
  Subtract3 : Sum  Inputs=+-
  Subtract4 : Sum  Inputs=+-
  q1_command : Outport
  q2_command : Outport  Port=2
  q3_command : Outport  Port=3
  wires:
  Saturation3/1 -> q3_command/1
  Subtract4/1 -> Custom Discrete PD (Wrist)/1(ey)
  Custom Discrete PD (Shoulder)/1(Fx) -> Saturation/1
  Custom Discrete PD (Elbow)/1(Fy) -> Saturation1/1
  Saturation/1 -> q1_command/1
  Subtract2/1 -> Custom Discrete PD (Shoulder)/1(ex)
  Saturation1/1 -> q2_command/1
  Custom Discrete PD (Wrist)/1(Fy) -> Saturation3/1
  Subtract3/1 -> Custom Discrete PD (Elbow)/1(ey)
  Data Store Read/1 -> Subtract2/2
  Data Store Read5/1 -> Subtract3/2
  Data Store Read6/1 -> Subtract4/2
  q1_desired/1 -> Subtract2/1
  q2_desired/1 -> Subtract3/1
  q3_desired/1 -> Subtract4/1

== system MPCfastmpc/PhaseSpace Camera Code/Use Hardware to Obtain States/Adjust Time/Enabled Subsystem ==
  In1 : Inport
  Enable : EnablePort
  Memory : Memory
  Out1 : Outport
  wires:
  Memory/1 -> Out1/1
  In1/1 -> Memory/1

== system MPCfastmpc/PhaseSpace Camera Code/Use Hardware to Obtain States/Adjust Time/Enabled Subsystem1 ==
  In2 : Inport
  In1 : Inport  Port=2
  Enable : EnablePort
  Subtract : Sum  Inputs=+-
  Out1 : Outport
  wires:
  Subtract/1 -> Out1/1
  In1/1 -> Subtract/1
  In2/1 -> Subtract/2

== system MPCfastmpc/PhaseSpace Camera Code/Use Hardware to Obtain States/x_dot -> x1/Hold this value ==
  In1 : Inport
  Action Port : ActionPort  ActionPortLabel=if(u1 ~= 0)
  Out1 : Outport  VectorParamsAs1DForOutWhenUnconnected=off
  wires:
  In1/1 -> Out1/1

== system MPCfastmpc/PhaseSpace Camera Code/Use Hardware to Obtain States/x_dot -> x10/Hold this value ==
  In1 : Inport
  Action Port : ActionPort  ActionPortLabel=if(u1 ~= 0)
  Out1 : Outport  VectorParamsAs1DForOutWhenUnconnected=off
  wires:
  In1/1 -> Out1/1

== system MPCfastmpc/PhaseSpace Camera Code/Use Hardware to Obtain States/x_dot -> x11/Hold this value ==
  In1 : Inport
  Action Port : ActionPort  ActionPortLabel=if(u1 ~= 0)
  Out1 : Outport  VectorParamsAs1DForOutWhenUnconnected=off
  wires:
  In1/1 -> Out1/1

== system MPCfastmpc/PhaseSpace Camera Code/Use Hardware to Obtain States/x_dot -> x12/Hold this value ==
  In1 : Inport
  Action Port : ActionPort  ActionPortLabel=if(u1 ~= 0)
  Out1 : Outport  VectorParamsAs1DForOutWhenUnconnected=off
  wires:
  In1/1 -> Out1/1

== system MPCfastmpc/PhaseSpace Camera Code/Use Hardware to Obtain States/x_dot -> x13/Hold this value ==
  In1 : Inport
  Action Port : ActionPort  ActionPortLabel=if(u1 ~= 0)
  Out1 : Outport  VectorParamsAs1DForOutWhenUnconnected=off
  wires:
  In1/1 -> Out1/1

== system MPCfastmpc/PhaseSpace Camera Code/Use Hardware to Obtain States/x_dot -> x14/Hold this value ==
  In1 : Inport
  Action Port : ActionPort  ActionPortLabel=if(u1 ~= 0)
  Out1 : Outport  VectorParamsAs1DForOutWhenUnconnected=off
  wires:
  In1/1 -> Out1/1

== system MPCfastmpc/PhaseSpace Camera Code/Use Hardware to Obtain States/x_dot -> x15/Hold this value ==
  In1 : Inport
  Action Port : ActionPort  ActionPortLabel=if(u1 ~= 0)
  Out1 : Outport  VectorParamsAs1DForOutWhenUnconnected=off
  wires:
  In1/1 -> Out1/1

== system MPCfastmpc/PhaseSpace Camera Code/Use Hardware to Obtain States/x_dot -> x16/Hold this value ==
  In1 : Inport
  Action Port : ActionPort  ActionPortLabel=if(u1 ~= 0)
  Out1 : Outport  VectorParamsAs1DForOutWhenUnconnected=off
  wires:
  In1/1 -> Out1/1

== system MPCfastmpc/PhaseSpace Camera Code/Use Hardware to Obtain States/x_dot -> x17/Hold this value ==
  In1 : Inport
  Action Port : ActionPort  ActionPortLabel=if(u1 ~= 0)
  Out1 : Outport  VectorParamsAs1DForOutWhenUnconnected=off
  wires:
  In1/1 -> Out1/1

== system MPCfastmpc/PhaseSpace Camera Code/Use Hardware to Obtain States/x_dot -> x18/Hold this value ==
  In1 : Inport
  Action Port : ActionPort  ActionPortLabel=if(u1 ~= 0)
  Out1 : Outport  VectorParamsAs1DForOutWhenUnconnected=off
  wires:
  In1/1 -> Out1/1

== system MPCfastmpc/PhaseSpace Camera Code/Use Hardware to Obtain States/x_dot -> x2/Hold this value ==
  In1 : Inport
  Action Port : ActionPort  ActionPortLabel=if(u1 ~= 0)
  Out1 : Outport  VectorParamsAs1DForOutWhenUnconnected=off
  wires:
  In1/1 -> Out1/1

== system MPCfastmpc/PhaseSpace Camera Code/Use Hardware to Obtain States/x_dot -> x3/Hold this value ==
  In1 : Inport
  Action Port : ActionPort  ActionPortLabel=if(u1 ~= 0)
  Out1 : Outport  VectorParamsAs1DForOutWhenUnconnected=off
  wires:
  In1/1 -> Out1/1

== system MPCfastmpc/PhaseSpace Camera Code/Use Hardware to Obtain States/x_dot -> x4/Hold this value ==
  In1 : Inport
  Action Port : ActionPort  ActionPortLabel=if(u1 ~= 0)
  Out1 : Outport  VectorParamsAs1DForOutWhenUnconnected=off
  wires:
  In1/1 -> Out1/1

== system MPCfastmpc/PhaseSpace Camera Code/Use Hardware to Obtain States/x_dot -> x5/Hold this value ==
  In1 : Inport
  Action Port : ActionPort  ActionPortLabel=if(u1 ~= 0)
  Out1 : Outport  VectorParamsAs1DForOutWhenUnconnected=off
  wires:
  In1/1 -> Out1/1

== system MPCfastmpc/PhaseSpace Camera Code/Use Hardware to Obtain States/x_dot -> x6/Hold this value ==
  In1 : Inport
  Action Port : ActionPort  ActionPortLabel=if(u1 ~= 0)
  Out1 : Outport  VectorParamsAs1DForOutWhenUnconnected=off
  wires:
  In1/1 -> Out1/1

== system MPCfastmpc/PhaseSpace Camera Code/Use Hardware to Obtain States/x_dot -> x7/Hold this value ==
  In1 : Inport
  Action Port : ActionPort  ActionPortLabel=if(u1 ~= 0)
  Out1 : Outport  VectorParamsAs1DForOutWhenUnconnected=off
  wires:
  In1/1 -> Out1/1

== system MPCfastmpc/PhaseSpace Camera Code/Use Hardware to Obtain States/x_dot -> x8/Hold this value ==
  In1 : Inport
  Action Port : ActionPort  ActionPortLabel=if(u1 ~= 0)
  Out1 : Outport  VectorParamsAs1DForOutWhenUnconnected=off
  wires:
  In1/1 -> Out1/1

== system MPCfastmpc/PhaseSpace Camera Code/Use Hardware to Obtain States/x_dot -> x9/Hold this value ==
  In1 : Inport
  Action Port : ActionPort  ActionPortLabel=if(u1 ~= 0)
  Out1 : Outport  VectorParamsAs1DForOutWhenUnconnected=off
  wires:
  In1/1 -> Out1/1

== system MPCfastmpc/Simulate Plant Dynamics/BLACK Dynamics/x_dot -> x1/Hold this value ==
  In1 : Inport
  Action Port : ActionPort  ActionPortLabel=if(u1 ~= 0)
  Out1 : Outport  VectorParamsAs1DForOutWhenUnconnected=off
  wires:
  In1/1 -> Out1/1

== system MPCfastmpc/Simulate Plant Dynamics/BLACK Dynamics/x_dot -> x2/Hold this value ==
  In1 : Inport
  Action Port : ActionPort  ActionPortLabel=if(u1 ~= 0)
  Out1 : Outport  VectorParamsAs1DForOutWhenUnconnected=off
  wires:
  In1/1 -> Out1/1

== system MPCfastmpc/Simulate Plant Dynamics/BLACK Dynamics/x_dot -> x3/Hold this value ==
  In1 : Inport
  Action Port : ActionPort  ActionPortLabel=if(u1 ~= 0)
  Out1 : Outport  VectorParamsAs1DForOutWhenUnconnected=off
  wires:
  In1/1 -> Out1/1

== system MPCfastmpc/Simulate Plant Dynamics/BLACK Dynamics/x_dot -> x4/Hold this value ==
  In1 : Inport
  Action Port : ActionPort  ActionPortLabel=if(u1 ~= 0)
  Out1 : Outport  VectorParamsAs1DForOutWhenUnconnected=off
  wires:
  In1/1 -> Out1/1

== system MPCfastmpc/Simulate Plant Dynamics/BLACK Dynamics/x_dot -> x7/Hold this value ==
  In1 : Inport
  Action Port : ActionPort  ActionPortLabel=if(u1 ~= 0)
  Out1 : Outport  VectorParamsAs1DForOutWhenUnconnected=off
  wires:
  In1/1 -> Out1/1

== system MPCfastmpc/Simulate Plant Dynamics/BLUE Dynamics/x_dot -> x1/Hold this value ==
  In1 : Inport
  Action Port : ActionPort  ActionPortLabel=if(u1 ~= 0)
  Out1 : Outport  VectorParamsAs1DForOutWhenUnconnected=off
  wires:
  In1/1 -> Out1/1

== system MPCfastmpc/Simulate Plant Dynamics/BLUE Dynamics/x_dot -> x2/Hold this value ==
  In1 : Inport
  Action Port : ActionPort  ActionPortLabel=if(u1 ~= 0)
  Out1 : Outport  VectorParamsAs1DForOutWhenUnconnected=off
  wires:
  In1/1 -> Out1/1

== system MPCfastmpc/Simulate Plant Dynamics/BLUE Dynamics/x_dot -> x3/Hold this value ==
  In1 : Inport
  Action Port : ActionPort  ActionPortLabel=if(u1 ~= 0)
  Out1 : Outport  VectorParamsAs1DForOutWhenUnconnected=off
  wires:
  In1/1 -> Out1/1

== system MPCfastmpc/Simulate Plant Dynamics/BLUE Dynamics/x_dot -> x4/Hold this value ==
  In1 : Inport
  Action Port : ActionPort  ActionPortLabel=if(u1 ~= 0)
  Out1 : Outport  VectorParamsAs1DForOutWhenUnconnected=off
  wires:
  In1/1 -> Out1/1

== system MPCfastmpc/Simulate Plant Dynamics/BLUE Dynamics/x_dot -> x7/Hold this value ==
  In1 : Inport
  Action Port : ActionPort  ActionPortLabel=if(u1 ~= 0)
  Out1 : Outport  VectorParamsAs1DForOutWhenUnconnected=off
  wires:
  In1/1 -> Out1/1

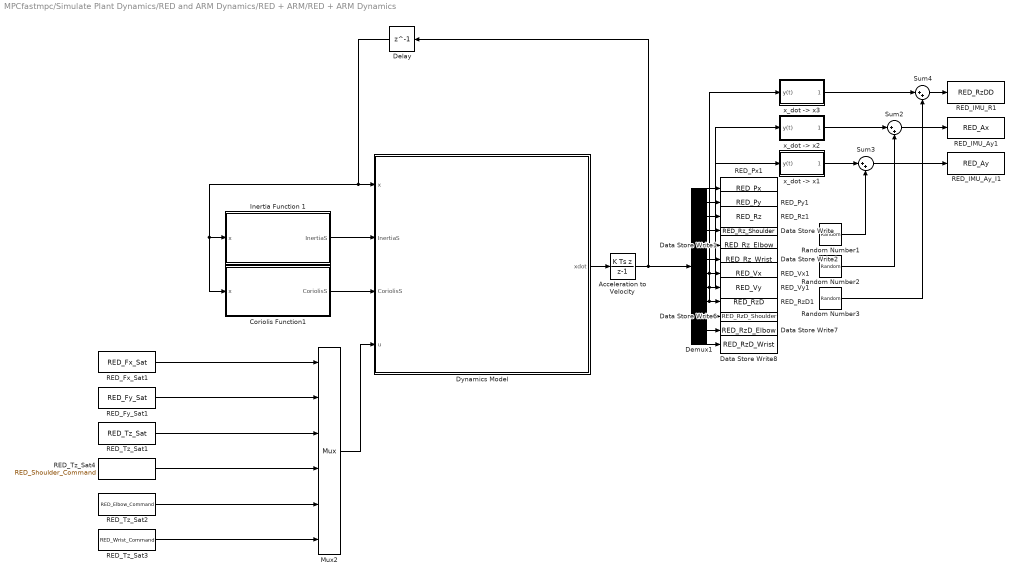
== system MPCfastmpc/Simulate Plant Dynamics/RED and ARM Dynamics/RED + ARM/RED + ARM Dynamics ==
  Acceleration to Velocity : DiscreteIntegrator  IntegratorMethod=Integration: Backward Euler  InitialCondition=[drop_states_RED,drop_states_ARM,0,0,0,0,0,0]  SampleTime=-1  ICPrevOutput=DiscIntNeverNeededParam  ICPrevScaledInput=DiscIntNeverNeededParam
  Coriolis Function1 : MATLAB Function  TreatAsAtomicUnit=on
  Data Store Write : DataStoreWrite  DataStoreName=RED_Rz_Shoulder  IndexOptions=Index vector (dialog)  Indices=1  OutputSizes=1
  Data Store Write1 : DataStoreWrite  DataStoreName=RED_Rz_Elbow  IndexOptions=Index vector (dialog)  Indices=1  OutputSizes=1
  Data Store Write2 : DataStoreWrite  DataStoreName=RED_Rz_Wrist  IndexOptions=Index vector (dialog)  Indices=1  OutputSizes=1
  Data Store Write6 : DataStoreWrite  DataStoreName=RED_RzD_Shoulder  IndexOptions=Index vector (dialog)  Indices=1  OutputSizes=1
  Data Store Write7 : DataStoreWrite  DataStoreName=RED_RzD_Elbow  IndexOptions=Index vector (dialog)  Indices=1  OutputSizes=1
  Data Store Write8 : DataStoreWrite  DataStoreName=RED_RzD_Wrist  IndexOptions=Index vector (dialog)  Indices=1  OutputSizes=1
  Delay : Delay  DelayLength=1
  Demux1 : Demux  Outputs=12
  Dynamics Model : MATLAB Function  TreatAsAtomicUnit=on
  Inertia Function 1 : MATLAB Function  TreatAsAtomicUnit=on
  Mux2 : Mux  Inputs=6
  RED_Fx_Sat1 : DataStoreRead  DataStoreName=RED_Fx_Sat  IndexOptions=Index vector (dialog)  Indices=1  OutputSizes=1
  RED_Fy_Sat1 : DataStoreRead  DataStoreName=RED_Fy_Sat  IndexOptions=Index vector (dialog)  Indices=1  OutputSizes=1
  RED_IMU_Ay1 : DataStoreWrite  DataStoreName=RED_Ax  IndexOptions=Index vector (dialog)  Indices=1  OutputSizes=1
  RED_IMU_Ay_I1 : DataStoreWrite  DataStoreName=RED_Ay  IndexOptions=Index vector (dialog)  Indices=1  OutputSizes=1
  RED_IMU_R1 : DataStoreWrite  DataStoreName=RED_RzDD  IndexOptions=Index vector (dialog)  Indices=1  OutputSizes=1
  RED_Px1 : DataStoreWrite  DataStoreName=RED_Px  IndexOptions=Index vector (dialog)  Indices=1  OutputSizes=1
  RED_Py1 : DataStoreWrite  DataStoreName=RED_Py  IndexOptions=Index vector (dialog)  Indices=1  OutputSizes=1
  RED_Rz1 : DataStoreWrite  DataStoreName=RED_Rz  IndexOptions=Index vector (dialog)  Indices=1  OutputSizes=1
  RED_RzD1 : DataStoreWrite  DataStoreName=RED_RzD  IndexOptions=Index vector (dialog)  Indices=1  OutputSizes=1
  RED_Tz_Sat1 : DataStoreRead  DataStoreName=RED_Tz_Sat  IndexOptions=Index vector (dialog)  Indices=1  OutputSizes=1
  RED_Tz_Sat2 : DataStoreRead  DataStoreName=RED_Elbow_Command  IndexOptions=Index vector (dialog)  Indices=1  OutputSizes=1
  RED_Tz_Sat3 : DataStoreRead  DataStoreName=RED_Wrist_Command  IndexOptions=Index vector (dialog)  Indices=1  OutputSizes=1
  RED_Tz_Sat4 : DataStoreRead  DataStoreName=RED_Shoulder_Command  IndexOptions=Index vector (dialog)  Indices=1  OutputSizes=1
  RED_Vx1 : DataStoreWrite  DataStoreName=RED_Vx  IndexOptions=Index vector (dialog)  Indices=1  OutputSizes=1
  RED_Vy1 : DataStoreWrite  DataStoreName=RED_Vy  IndexOptions=Index vector (dialog)  Indices=1  OutputSizes=1
  Random Number1 : RandomNumber  Variance=0
  Random Number2 : RandomNumber  Variance=0
  Random Number3 : RandomNumber  Variance=0
  Sum2 : Sum  Inputs=|++
  Sum3 : Sum  Inputs=|++
  Sum4 : Sum  Inputs=|++
  "x_dot -> x1" : Subsystem
  "x_dot -> x2" : Subsystem
  "x_dot -> x3" : Subsystem
  wires:
  Demux1/2 -> RED_Py1/1
  Random Number1/1 -> Sum3/2
  Random Number2/1 -> Sum2/2
  Demux1/3 -> RED_Rz1/1
  Demux1/9 -> "x_dot -> x3"/1(y(t)), RED_RzD1/1
  RED_Tz_Sat1/1 -> Mux2/3
  Delay/1 -> Dynamics Model/1(x), Coriolis Function1/1(x), Inertia Function 1/1(x)
  RED_Fx_Sat1/1 -> Mux2/1
  "x_dot -> x1"/1(dy(t)/dt) -> Sum3/1
  Demux1/8 -> "x_dot -> x1"/1(y(t)), RED_Vy1/1
  Demux1/1 -> RED_Px1/1
  "x_dot -> x2"/1(dy(t)/dt) -> Sum2/1
  Random Number3/1 -> Sum4/2
  Mux2/1 -> Dynamics Model/4(u)
  Demux1/7 -> "x_dot -> x2"/1(y(t)), RED_Vx1/1
  Demux1/12 -> Data Store Write8/1
  Inertia Function 1/1(InertiaS) -> Dynamics Model/2(InertiaS)
  Demux1/11 -> Data Store Write7/1
  Sum2/1 -> RED_IMU_Ay1/1
  Sum4/1 -> RED_IMU_R1/1
  Acceleration to Velocity/1 -> Delay/1, Demux1/1
  Dynamics Model/1(xdot) -> Acceleration to Velocity/1
  Demux1/10 -> Data Store Write6/1
  Demux1/5 -> Data Store Write1/1
  Coriolis Function1/1(CoriolisS) -> Dynamics Model/3(CoriolisS)
  Demux1/6 -> Data Store Write2/1
  Sum3/1 -> RED_IMU_Ay_I1/1
  Demux1/4 -> Data Store Write/1
  RED_Fy_Sat1/1 -> Mux2/2
  "x_dot -> x3"/1(dy(t)/dt) -> Sum4/1
  RED_Tz_Sat4/1 -> Mux2/4
  RED_Tz_Sat2/1 -> Mux2/5
  RED_Tz_Sat3/1 -> Mux2/6

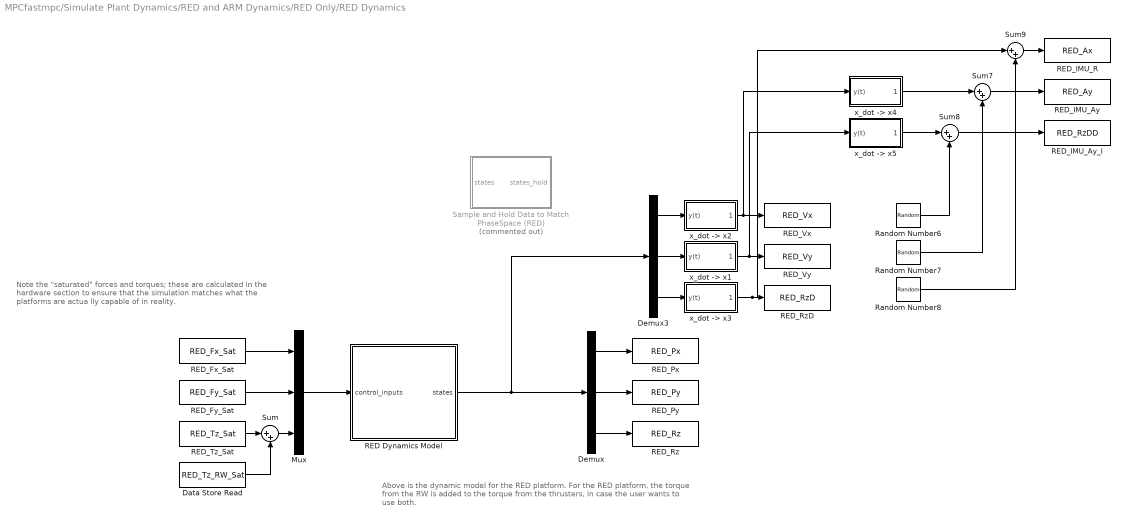
== system MPCfastmpc/Simulate Plant Dynamics/RED and ARM Dynamics/RED Only/RED Dynamics ==
  note: Above is the dynamic model for the RED
      | platform. For the RED platform, the torque from the RW is added to the torque from the thrusters, in case the user wants to use both.
  note: Note the "saturated" forces and torques; these are calculated in the hardware section to ensure that the simulation matches what the platforms are actua lly capable of in reality.
  Data Store Read : DataStoreRead  DataStoreName=RED_Tz_RW_Sat  IndexOptions=Index vector (dialog)  Indices=1  OutputSizes=1
  Demux : Demux  Outputs=3
  Demux3 : Demux  Outputs=3
  Mux : Mux  Inputs=3
  RED Dynamics Model : Subsystem  SystemSampleTime=serverRate
  RED_Fx_Sat : DataStoreRead  DataStoreName=RED_Fx_Sat  IndexOptions=Index vector (dialog)  Indices=1  OutputSizes=1
  RED_Fy_Sat : DataStoreRead  DataStoreName=RED_Fy_Sat  IndexOptions=Index vector (dialog)  Indices=1  OutputSizes=1
  RED_IMU_Ay : DataStoreWrite  DataStoreName=RED_Ay  IndexOptions=Index vector (dialog)  Indices=1  OutputSizes=1
  RED_IMU_Ay_I : DataStoreWrite  DataStoreName=RED_RzDD  IndexOptions=Index vector (dialog)  Indices=1  OutputSizes=1
  RED_IMU_R : DataStoreWrite  DataStoreName=RED_Ax  IndexOptions=Index vector (dialog)  Indices=1  OutputSizes=1
  RED_Px : DataStoreWrite  DataStoreName=RED_Px  IndexOptions=Index vector (dialog)  Indices=1  OutputSizes=1
  RED_Py : DataStoreWrite  DataStoreName=RED_Py  IndexOptions=Index vector (dialog)  Indices=1  OutputSizes=1
  RED_Rz : DataStoreWrite  DataStoreName=RED_Rz  IndexOptions=Index vector (dialog)  Indices=1  OutputSizes=1
  RED_RzD : DataStoreWrite  DataStoreName=RED_RzD  IndexOptions=Index vector (dialog)  Indices=1  OutputSizes=1
  RED_Tz_Sat : DataStoreRead  DataStoreName=RED_Tz_Sat  IndexOptions=Index vector (dialog)  Indices=1  OutputSizes=1
  RED_Vx : DataStoreWrite  DataStoreName=RED_Vx  IndexOptions=Index vector (dialog)  Indices=1  OutputSizes=1
  RED_Vy : DataStoreWrite  DataStoreName=RED_Vy  IndexOptions=Index vector (dialog)  Indices=1  OutputSizes=1
  Random Number6 : RandomNumber  Variance=1.5e-6
  Random Number7 : RandomNumber  Variance=1.5e-6
  Random Number8 : RandomNumber  Variance=1.5e-6
  Sample and Hold Data to Match PhaseSpace (RED) : Subsystem  Commented=on
  Sum{,7..9} (4 alike) : Sum  Inputs=|++
  "x_dot -> x1" : Subsystem
  "x_dot -> x2" : Subsystem
  "x_dot -> x3" : Subsystem
  "x_dot -> x4" : Subsystem
  "x_dot -> x5" : Subsystem
  wires:
  Mux/1 -> RED Dynamics Model/1(control_inputs)
  Demux3/3 -> "x_dot -> x3"/1(y(t))
  "x_dot -> x2"/1(dy(t)/dt) -> "x_dot -> x4"/1(y(t)), RED_Vx/1
  Sum9/1 -> RED_IMU_R/1
  Demux3/2 -> "x_dot -> x1"/1(y(t))
  "x_dot -> x3"/1(dy(t)/dt) -> Sum9/1, RED_RzD/1
  RED_Fy_Sat/1 -> Mux/2
  RED_Fx_Sat/1 -> Mux/1
  Demux/1 -> RED_Px/1
  Sum/1 -> Mux/3
  Demux3/1 -> "x_dot -> x2"/1(y(t))
  "x_dot -> x1"/1(dy(t)/dt) -> "x_dot -> x5"/1(y(t)), RED_Vy/1
  Data Store Read/1 -> Sum/2
  "x_dot -> x4"/1(dy(t)/dt) -> Sum7/1
  Random Number7/1 -> Sum7/2
  "x_dot -> x5"/1(dy(t)/dt) -> Sum8/1
  Random Number8/1 -> Sum9/2
  Demux/2 -> RED_Py/1
  RED Dynamics Model/1(states) -> Demux3/1, Demux/1
  Demux/3 -> RED_Rz/1
  RED_Tz_Sat/1 -> Sum/1
  Sum7/1 -> RED_IMU_Ay/1
  Sum8/1 -> RED_IMU_Ay_I/1
  Random Number6/1 -> Sum8/2

== system MPCfastmpc/Thruster Control Code/Change BLACK Behavior/Calculate Thruster ON//OFF/Rotate Forces to Inertial ==
  "F_b " : Inport
  Rz : Inport  Port=2
  Create Rotation Matrix : MATLAB Function  TreatAsAtomicUnit=on
  Rotate F_b to F_I : Product  Multiplication=Matrix(*)
  F_I : Outport  VectorParamsAs1DForOutWhenUnconnected=off
  wires:
  "F_b "/1 -> Rotate F_b to F_I/2
  Rotate F_b to F_I/1 -> F_I/1
  Create Rotation Matrix/1(C_Ib) -> Rotate F_b to F_I/1
  Rz/1 -> Create Rotation Matrix/1(Rz)

== system MPCfastmpc/Thruster Control Code/Change BLACK Behavior/Calculate Thruster ON//OFF/pseudo-inverse ==
  H : Inport
  Product : Product  Multiplication=Matrix(*)
  Product1 : Product  Inputs=/  Multiplication=Matrix(*)
  Product2 : Product  Multiplication=Matrix(*)
  transpose : PermuteDimensions
  invH : Outport  VectorParamsAs1DForOutWhenUnconnected=off
  wires:
  Product2/1 -> invH/1
  transpose/1 -> Product/2, Product2/1
  Product/1 -> Product1/1
  H/1 -> Product/1, transpose/1
  Product1/1 -> Product2/2
